simulink model "VCU_CS75_12_27_test_log"  (R2014a)
settings: Solver=FixedStepDiscrete  StartTime=0.0  StopTime=25  FixedStep=0.0005  RelTol=1e-3
undefined symbols (not defined in the file or in its folder): ecucoder_acal, ErrorSumMax1, ErrorSumMax2, ErrorSumMax3, I1, I2, I3, I_SW01_L, LaterlAngleCommand, LDW, Log_ErrorSumMax1, Log_ErrorSumMax2, Log_I1, Log_I2, Log_P1, Log_P2, Log_Takeover, P1, P2, P3, RemoteAcc, RemoteAcclPosition
libraries: simulink x927, ec5744lib x40
(part 2 of 31)

== system VCU_CS75_12_27_test_log/长安CS75底盘程序，20ms一次/Input/CAN1_Rx/TCU_286 ==
  CANReceive : ec5744lib/RapidECU_U3/04CANCommunication/CANReceive  canmodule=1  canbuffer=22  canmessageid=hex2dec('286')  canmessagetype=Standard(11-bit ID)  datalength=8  sampletime=-1
  ReceiveMessages : Subsystem
  Terminator : Terminator
  Terminator1 : Terminator
  TCU_286 : Outport
  wires:
  ReceiveMessages/1(TCU_286) -> TCU_286/1
  CANReceive/3 -> Terminator/1
  CANReceive/4 -> ReceiveMessages/2(In2)
  CANReceive/1 -> ReceiveMessages/Trigger
  CANReceive/2 -> ReceiveMessages/1(In1)
  CANReceive/5 -> Terminator1/1

== system VCU_CS75_12_27_test_log/长安CS75底盘程序，20ms一次/Input/DBC转化的messages（存底）/ReceiveMessages ==
  EMS_205 : Subsystem
  EMS_205_GND : Ground
  EMS_CheckSum_205_Ter : Terminator
  EMS_ESPTorqReuestAvailability_Ter : Terminator
  EMS_FrictionalTorq_Ter : Terminator
  EMS_IndicatedDriverReqTorq_Ter : Terminator
  EMS_IndicatedRealEngTorq_Ter : Terminator
  EMS_RollingCounter_id205_Ter : Terminator
  EMS_TorqFailure_Ter : Terminator
  wires:
  EMS_205/1(EMS_ESPTorqReuestAvailability_Out) -> EMS_ESPTorqReuestAvailability_Ter/1
  EMS_205/2(EMS_TorqFailure_Out) -> EMS_TorqFailure_Ter/1
  EMS_205/3(EMS_IndicatedDriverReqTorq_Out) -> EMS_IndicatedDriverReqTorq_Ter/1
  EMS_205/4(EMS_FrictionalTorq_Out) -> EMS_FrictionalTorq_Ter/1
  EMS_205/5(EMS_IndicatedRealEngTorq_Out) -> EMS_IndicatedRealEngTorq_Ter/1
  EMS_205/6(EMS_RollingCounter_id205_Out) -> EMS_RollingCounter_id205_Ter/1
  EMS_205/7(EMS_CheckSum_205_Out) -> EMS_CheckSum_205_Ter/1
  EMS_205_GND/1 -> EMS_205/1(input)

== system VCU_CS75_12_27_test_log/长安CS75底盘程序，20ms一次/Input/DBC转化的messages（存底）/ReceiveMessages1 ==
  EMS_255 : Subsystem
  EMS_255_GND : Ground
  EMS_AccPedal_Ter : Terminator
  EMS_AccpedelError_Ter : Terminator
  EMS_BrakePedalStatus_Ter : Terminator
  EMS_CheckSum_255_Ter : Terminator
  EMS_EngineSpeedError_Ter : Terminator
  EMS_EngineSpeed_Ter : Terminator
  EMS_RollingCounter_id255_Ter : Terminator
  wires:
  EMS_255/1(EMS_BrakePedalStatus_Out) -> EMS_BrakePedalStatus_Ter/1
  EMS_255/2(EMS_AccpedelError_Out) -> EMS_AccpedelError_Ter/1
  EMS_255/3(EMS_EngineSpeedError_Out) -> EMS_EngineSpeedError_Ter/1
  EMS_255/4(EMS_EngineSpeed_Out) -> EMS_EngineSpeed_Ter/1
  EMS_255/5(EMS_AccPedal_Out) -> EMS_AccPedal_Ter/1
  EMS_255/6(EMS_RollingCounter_id255_Out) -> EMS_RollingCounter_id255_Ter/1
  EMS_255/7(EMS_CheckSum_255_Out) -> EMS_CheckSum_255_Ter/1
  EMS_255_GND/1 -> EMS_255/1(input)

== system VCU_CS75_12_27_test_log/长安CS75底盘程序，20ms一次/Input/DBC转化的messages（存底）/ReceiveMessages10 ==
  ESP_287 : Subsystem
  ESP_287_GND : Ground
  ESP_CheckSum_Ter : Terminator
  ESP_HBBActiveStatus_Ter : Terminator
  ESP_HBB_Status_Ter : Terminator
  ESP_HDC_Status_Ter : Terminator
  ESP_HHC_Available_Ter : Terminator
  ESP_LatAcceleration_Ter : Terminator
  ESP_LongAccelValid_Ter : Terminator
  ESP_LongAcceleration_Ter : Terminator
  ESP_RollingCounter_Ter : Terminator
  ESP_TODFastOpenRequest_Ter : Terminator
  ESP_TODTorqueMaxLimit_Ter : Terminator
  ESP_YawRate_Status_Ter : Terminator
  ESP_YawRate_Ter : Terminator
  wires:
  ESP_287_GND/1 -> ESP_287/1(input)
  ESP_287/13(ESP_RollingCounter_Out) -> ESP_RollingCounter_Ter/1
  ESP_287/12(ESP_CheckSum_Out) -> ESP_CheckSum_Ter/1
  ESP_287/11(ESP_YawRate_Status_Out) -> ESP_YawRate_Status_Ter/1
  ESP_287/10(ESP_LongAccelValid_Out) -> ESP_LongAccelValid_Ter/1
  ESP_287/9(ESP_HBBActiveStatus_Out) -> ESP_HBBActiveStatus_Ter/1
  ESP_287/8(ESP_HHC_Available_Out) -> ESP_HHC_Available_Ter/1
  ESP_287/7(ESP_HBB_Status_Out) -> ESP_HBB_Status_Ter/1
  ESP_287/6(ESP_YawRate_Out) -> ESP_YawRate_Ter/1
  ESP_287/5(ESP_LongAcceleration_Out) -> ESP_LongAcceleration_Ter/1
  ESP_287/4(ESP_LatAcceleration_Out) -> ESP_LatAcceleration_Ter/1
  ESP_287/3(ESP_TODFastOpenRequest_Out) -> ESP_TODFastOpenRequest_Ter/1
  ESP_287/2(ESP_HDC_Status_Out) -> ESP_HDC_Status_Ter/1
  ESP_287/1(ESP_TODTorqueMaxLimit_Out) -> ESP_TODTorqueMaxLimit_Ter/1

== system VCU_CS75_12_27_test_log/长安CS75底盘程序，20ms一次/Input/DBC转化的messages（存底）/ReceiveMessages11 ==
  HU_AEBOnOffSetting_Ter : Terminator
  HU_AEBSetting_551 : Subsystem
  HU_AEBSetting_551_GND : Ground
  HU_FCWSetting_Ter : Terminator
  HU_LCASetting_Ter : Terminator
  wires:
  HU_AEBSetting_551_GND/1 -> HU_AEBSetting_551/1(input)
  HU_AEBSetting_551/3(HU_FCWSetting_Out) -> HU_FCWSetting_Ter/1
  HU_AEBSetting_551/2(HU_LCASetting_Out) -> HU_LCASetting_Ter/1
  HU_AEBSetting_551/1(HU_AEBOnOffSetting_Out) -> HU_AEBOnOffSetting_Ter/1

== system VCU_CS75_12_27_test_log/长安CS75底盘程序，20ms一次/Input/DBC转化的messages（存底）/ReceiveMessages12 ==
  HU_AudioWarningEnable_Ter : Terminator
  HU_BSD_LCAEnable_Ter : Terminator
  HU_CTAEnable_Ter : Terminator
  HU_DSMMemoryPositionFeedback_Ter : Terminator
  HU_DVRBrowseCommand_Ter : Terminator
  HU_HMAEnable_Ter : Terminator
  HU_IACCEnable_Ter : Terminator
  HU_LASModeSelection_Ter : Terminator
  HU_LASSetting_0x541 : Subsystem
  HU_LASSetting_0x541_GND : Ground
  HU_LASWarningModeSelection_Ter : Terminator
  HU_LCATTCSetting_Ter : Terminator
  HU_LDWShakeLev_Ter : Terminator
  HU_LdwSensitivity_Ter : Terminator
  HU_LockCtrlEnable_Ter : Terminator
  HU_ObstacleSafeDistanceSet_Ter : Terminator
  HU_OverspeedSoundWarEnable_Ter : Terminator
  HU_OverspeedWarningEnable_Ter : Terminator
  HU_OverspeedWarningOffset_Ter : Terminator
  HU_ParkingConfirm_Ter : Terminator
  HU_ParkingResume_Ter : Terminator
  HU_RCWEnable_Ter : Terminator
  HU_RCWSoundEnable_Ter : Terminator
  HU_RemoteDistanceSet_Ter : Terminator
  HU_SEWEnable_Ter : Terminator
  HU_SLASwitch_Ter : Terminator
  HU_Uls_BSD_Activation_Ter : Terminator
  HU_Uls_FKP_Activation_Ter : Terminator
  wires:
  HU_LASSetting_0x541_GND/1 -> HU_LASSetting_0x541/1(input)
  HU_LASSetting_0x541/26(HU_DVRBrowseCommand_Out) -> HU_DVRBrowseCommand_Ter/1
  HU_LASSetting_0x541/25(HU_ObstacleSafeDistanceSet_Out) -> HU_ObstacleSafeDistanceSet_Ter/1
  HU_LASSetting_0x541/24(HU_ParkingConfirm_Out) -> HU_ParkingConfirm_Ter/1
  HU_LASSetting_0x541/23(HU_RemoteDistanceSet_Out) -> HU_RemoteDistanceSet_Ter/1
  HU_LASSetting_0x541/22(HU_DSMMemoryPositionFeedback_Out) -> HU_DSMMemoryPositionFeedback_Ter/1
  HU_LASSetting_0x541/21(HU_ParkingResume_Out) -> HU_ParkingResume_Ter/1
  HU_LASSetting_0x541/20(HU_Uls_FKP_Activation_Out) -> HU_Uls_FKP_Activation_Ter/1
  HU_LASSetting_0x541/19(HU_LCATTCSetting_Out) -> HU_LCATTCSetting_Ter/1
  HU_LASSetting_0x541/18(HU_Uls_BSD_Activation_Out) -> HU_Uls_BSD_Activation_Ter/1
  HU_LASSetting_0x541/17(HU_OverspeedWarningOffset_Out) -> HU_OverspeedWarningOffset_Ter/1
  HU_LASSetting_0x541/16(HU_OverspeedWarningEnable_Out) -> HU_OverspeedWarningEnable_Ter/1
  HU_LASSetting_0x541/15(HU_OverspeedSoundWarEnable_Out) -> HU_OverspeedSoundWarEnable_Ter/1
  HU_LASSetting_0x541/14(HU_IACCEnable_Out) -> HU_IACCEnable_Ter/1
  HU_LASSetting_0x541/13(HU_LockCtrlEnable_Out) -> HU_LockCtrlEnable_Ter/1
  HU_LASSetting_0x541/12(HU_AudioWarningEnable_Out) -> HU_AudioWarningEnable_Ter/1
  HU_LASSetting_0x541/11(HU_LDWShakeLev_Out) -> HU_LDWShakeLev_Ter/1
  HU_LASSetting_0x541/10(HU_RCWSoundEnable_Out) -> HU_RCWSoundEnable_Ter/1
  HU_LASSetting_0x541/9(HU_SEWEnable_Out) -> HU_SEWEnable_Ter/1
  HU_LASSetting_0x541/8(HU_RCWEnable_Out) -> HU_RCWEnable_Ter/1
  HU_LASSetting_0x541/7(HU_HMAEnable_Out) -> HU_HMAEnable_Ter/1
  HU_LASSetting_0x541/6(HU_SLASwitch_Out) -> HU_SLASwitch_Ter/1
  HU_LASSetting_0x541/5(HU_LASWarningModeSelection_Out) -> HU_LASWarningModeSelection_Ter/1
  HU_LASSetting_0x541/4(HU_LdwSensitivity_Out) -> HU_LdwSensitivity_Ter/1
  HU_LASSetting_0x541/3(HU_LASModeSelection_Out) -> HU_LASModeSelection_Ter/1
  HU_LASSetting_0x541/2(HU_BSD_LCAEnable_Out) -> HU_BSD_LCAEnable_Ter/1
  HU_LASSetting_0x541/1(HU_CTAEnable_Out) -> HU_CTAEnable_Ter/1

== system VCU_CS75_12_27_test_log/长安CS75底盘程序，20ms一次/Input/DBC转化的messages（存底）/ReceiveMessages13 ==
  SAS_108 : Subsystem
  SAS_108_GND : Ground
  SAS_CRCCheck_Ter : Terminator
  SAS_Calibrated_Ter : Terminator
  SAS_RollingCounter_Ter : Terminator
  SAS_SASFailure_Ter : Terminator
  SAS_SteeringAngleSpeed_Ter : Terminator
  SAS_SteeringAngleValid_Ter : Terminator
  SAS_SteeringAngle_Ter : Terminator
  wires:
  SAS_108_GND/1 -> SAS_108/1(input)
  SAS_108/7(SAS_CRCCheck_Out) -> SAS_CRCCheck_Ter/1
  SAS_108/6(SAS_RollingCounter_Out) -> SAS_RollingCounter_Ter/1
  SAS_108/5(SAS_SteeringAngleValid_Out) -> SAS_SteeringAngleValid_Ter/1
  SAS_108/4(SAS_SASFailure_Out) -> SAS_SASFailure_Ter/1
  SAS_108/3(SAS_Calibrated_Out) -> SAS_Calibrated_Ter/1
  SAS_108/2(SAS_SteeringAngleSpeed_Out) -> SAS_SteeringAngleSpeed_Ter/1
  SAS_108/1(SAS_SteeringAngle_Out) -> SAS_SteeringAngle_Ter/1

== system VCU_CS75_12_27_test_log/长安CS75底盘程序，20ms一次/Input/DBC转化的messages（存底）/ReceiveMessages14 ==
  SCM_3B8 : Subsystem
  SCM_3B8_GND : Ground
  SCM_ACCCancel_Ter : Terminator
  SCM_ACCOn_Ter : Terminator
  SCM_IACCOn_Ter : Terminator
  SCM_Resume_Ter : Terminator
  SCM_Speeddecrease_Ter : Terminator
  SCM_TimeGap_Ter : Terminator
  wires:
  SCM_3B8_GND/1 -> SCM_3B8/1(input)
  SCM_3B8/6(SCM_IACCOn_Out) -> SCM_IACCOn_Ter/1
  SCM_3B8/5(SCM_TimeGap_Out) -> SCM_TimeGap_Ter/1
  SCM_3B8/4(SCM_Speeddecrease_Out) -> SCM_Speeddecrease_Ter/1
  SCM_3B8/3(SCM_Resume_Out) -> SCM_Resume_Ter/1
  SCM_3B8/2(SCM_ACCCancel_Out) -> SCM_ACCCancel_Ter/1
  SCM_3B8/1(SCM_ACCOn_Out) -> SCM_ACCOn_Ter/1

== system VCU_CS75_12_27_test_log/长安CS75底盘程序，20ms一次/Input/DBC转化的messages（存底）/ReceiveMessages15 ==
  SRS_005 : Subsystem
  SRS_005_GND : Ground
  SRS_DriverBuckleSwitchStatus_Ter : Terminator
  SRS_RollingCounter_Ter : Terminator
  wires:
  SRS_005_GND/1 -> SRS_005/1(input)
  SRS_005/2(SRS_RollingCounter_Out) -> SRS_RollingCounter_Ter/1
  SRS_005/1(SRS_DriverBuckleSwitchStatus_Out) -> SRS_DriverBuckleSwitchStatus_Ter/1

== system VCU_CS75_12_27_test_log/长安CS75底盘程序，20ms一次/Input/DBC转化的messages（存底）/ReceiveMessages16 ==
  TCU_286 : Subsystem
  TCU_286_GND : Ground
  TCU_ActualGearValid_Ter : Terminator
  TCU_ActualGear_Ter : Terminator
  TCU_GearShiftPosition_Ter : Terminator
  TCU_ShiftPositionValid_Ter : Terminator
  wires:
  TCU_286_GND/1 -> TCU_286/1(input)
  TCU_286/4(TCU_GearShiftPosition_Out) -> TCU_GearShiftPosition_Ter/1
  TCU_286/3(TCU_ActualGearValid_Out) -> TCU_ActualGearValid_Ter/1
  TCU_286/2(TCU_ShiftPositionValid_Out) -> TCU_ShiftPositionValid_Ter/1
  TCU_286/1(TCU_ActualGear_Out) -> TCU_ActualGear_Ter/1

== system VCU_CS75_12_27_test_log/长安CS75底盘程序，20ms一次/Input/DBC转化的messages（存底）/ReceiveMessages17 ==
  BCM_288 : Subsystem
  BCM_288_GND : Ground
  BCM_BuzzerWarningMode_Ter : Terminator
  BCM_DriverDoorLockStatus_Ter : Terminator
  BCM_DriverDoorStatus_Ter : Terminator
  BCM_FrontWashStatus_Ter : Terminator
  BCM_FrontWiperStatus_Ter : Terminator
  BCM_HoodStatus_Ter : Terminator
  BCM_LatchOverheatProtect_Ter : Terminator
  BCM_LeftRearDoorStatus_Ter : Terminator
  BCM_PassengerDoorLockStatus_Ter : Terminator
  BCM_PassengerDoorStatus_Ter : Terminator
  BCM_PowerStatusFeedback_Ter : Terminator
  BCM_RearWiperStatus_Ter : Terminator
  BCM_ReversePosition_Ter : Terminator
  BCM_RightRearDoorStatus_Ter : Terminator
  BCM_SystemFailureFlag_Ter : Terminator
  BCM_TrunkDoorStatus_Ter : Terminator
  BCM_TurnIndicatorLeft_Ter : Terminator
  BCM_TurnIndicatorRight_Ter : Terminator
  BCM_TurnLightSwitchSts_Ter : Terminator
  BCM_emergencylightstatus_Ter : Terminator
  wires:
  BCM_288_GND/1 -> BCM_288/1(input)
  BCM_288/20(BCM_LatchOverheatProtect_Out) -> BCM_LatchOverheatProtect_Ter/1
  BCM_288/19(BCM_SystemFailureFlag_Out) -> BCM_SystemFailureFlag_Ter/1
  BCM_288/18(BCM_BuzzerWarningMode_Out) -> BCM_BuzzerWarningMode_Ter/1
  BCM_288/17(BCM_TurnLightSwitchSts_Out) -> BCM_TurnLightSwitchSts_Ter/1
  BCM_288/16(BCM_ReversePosition_Out) -> BCM_ReversePosition_Ter/1
  BCM_288/15(BCM_FrontWiperStatus_Out) -> BCM_FrontWiperStatus_Ter/1
  BCM_288/14(BCM_RearWiperStatus_Out) -> BCM_RearWiperStatus_Ter/1
  BCM_288/13(BCM_PowerStatusFeedback_Out) -> BCM_PowerStatusFeedback_Ter/1
  BCM_288/12(BCM_DriverDoorLockStatus_Out) -> BCM_DriverDoorLockStatus_Ter/1
  BCM_288/11(BCM_emergencylightstatus_Out) -> BCM_emergencylightstatus_Ter/1
  BCM_288/10(BCM_PassengerDoorLockStatus_Out) -> BCM_PassengerDoorLockStatus_Ter/1
  BCM_288/9(BCM_DriverDoorStatus_Out) -> BCM_DriverDoorStatus_Ter/1
  BCM_288/8(BCM_PassengerDoorStatus_Out) -> BCM_PassengerDoorStatus_Ter/1
  BCM_288/7(BCM_LeftRearDoorStatus_Out) -> BCM_LeftRearDoorStatus_Ter/1
  BCM_288/6(BCM_RightRearDoorStatus_Out) -> BCM_RightRearDoorStatus_Ter/1
  BCM_288/5(BCM_TrunkDoorStatus_Out) -> BCM_TrunkDoorStatus_Ter/1
  BCM_288/4(BCM_HoodStatus_Out) -> BCM_HoodStatus_Ter/1
  BCM_288/3(BCM_TurnIndicatorLeft_Out) -> BCM_TurnIndicatorLeft_Ter/1
  BCM_288/2(BCM_TurnIndicatorRight_Out) -> BCM_TurnIndicatorRight_Ter/1
  BCM_288/1(BCM_FrontWashStatus_Out) -> BCM_FrontWashStatus_Ter/1

== system VCU_CS75_12_27_test_log/长安CS75底盘程序，20ms一次/Input/DBC转化的messages（存底）/ReceiveMessages18 ==
  BCM_328 : Subsystem
  BCM_328_GND : Ground
  LCM_DRLSts_Ter : Terminator
  LCM_DriveMode_Ter : Terminator
  LCM_LASSwitch_Ter : Terminator
  LCM_RearLeftTuningLightFaultSts_Ter : Terminator
  LCM_RearRightTuningLightFaultSts_Ter : Terminator
  LCM_ReverseLightSts_Ter : Terminator
  wires:
  BCM_328_GND/1 -> BCM_328/1(input)
  BCM_328/6(LCM_ReverseLightSts_Out) -> LCM_ReverseLightSts_Ter/1
  BCM_328/5(LCM_RearLeftTuningLightFaultSts_Out) -> LCM_RearLeftTuningLightFaultSts_Ter/1
  BCM_328/4(LCM_RearRightTuningLightFaultSts_Out) -> LCM_RearRightTuningLightFaultSts_Ter/1
  BCM_328/3(LCM_LASSwitch_Out) -> LCM_LASSwitch_Ter/1
  BCM_328/2(LCM_DRLSts_Out) -> LCM_DRLSts_Ter/1
  BCM_328/1(LCM_DriveMode_Out) -> LCM_DriveMode_Ter/1

== system VCU_CS75_12_27_test_log/长安CS75底盘程序，20ms一次/Input/DBC转化的messages（存底）/ReceiveMessages19 ==
  BCM_348 : Subsystem
  BCM_348_GND : Ground
  BCM_DriveMode_Ter : Terminator
  BCM_LockSignal_Ter : Terminator
  BCM_UnlockSignal_Ter : Terminator
  wires:
  BCM_348_GND/1 -> BCM_348/1(input)
  BCM_348/3(BCM_UnlockSignal_Out) -> BCM_UnlockSignal_Ter/1
  BCM_348/2(BCM_LockSignal_Out) -> BCM_LockSignal_Ter/1
  BCM_348/1(BCM_DriveMode_Out) -> BCM_DriveMode_Ter/1

== system VCU_CS75_12_27_test_log/长安CS75底盘程序，20ms一次/Input/DBC转化的messages（存底）/ReceiveMessages2 ==
  EMS_265 : Subsystem
  EMS_265_GND : Ground
  EMS_EngineStatus_Ter : Terminator
  EMS_FullLoadIndicatedTorq_Ter : Terminator
  EMS_RollingCounter_id265_Ter : Terminator
  EMS_TorqueConstant_Ter : Terminator
  wires:
  EMS_265/1(EMS_FullLoadIndicatedTorq_Out) -> EMS_FullLoadIndicatedTorq_Ter/1
  EMS_265/2(EMS_TorqueConstant_Out) -> EMS_TorqueConstant_Ter/1
  EMS_265/3(EMS_RollingCounter_id265_Out) -> EMS_RollingCounter_id265_Ter/1
  EMS_265/4(EMS_EngineStatus_Out) -> EMS_EngineStatus_Ter/1
  EMS_265_GND/1 -> EMS_265/1(input)

== system VCU_CS75_12_27_test_log/长安CS75底盘程序，20ms一次/Input/DBC转化的messages（存底）/ReceiveMessages20 ==
  BCM_3DF : Subsystem
  BCM_3DF_GND : Ground
  BCM_AmbientLightColorFeedback_Ter : Terminator
  BCM_CRC_Checksum_Ter : Terminator
  BCM_DriveModeFeedback_Ter : Terminator
  BCM_DriveModeStatus_Ter : Terminator
  BCM_DriveMode_Ter : Terminator
  BCM_EPSTorqueModeFeedback_Ter : Terminator
  BCM_EPSTorqueMode_Ter : Terminator
  BCM_RollingCounter_Ter : Terminator
  wires:
  BCM_3DF_GND/1 -> BCM_3DF/1(input)
  BCM_3DF/8(BCM_CRC_Checksum_Out) -> BCM_CRC_Checksum_Ter/1
  BCM_3DF/7(BCM_RollingCounter_Out) -> BCM_RollingCounter_Ter/1
  BCM_3DF/6(BCM_AmbientLightColorFeedback_Out) -> BCM_AmbientLightColorFeedback_Ter/1
  BCM_3DF/5(BCM_EPSTorqueModeFeedback_Out) -> BCM_EPSTorqueModeFeedback_Ter/1
  BCM_3DF/4(BCM_DriveModeFeedback_Out) -> BCM_DriveModeFeedback_Ter/1
  BCM_3DF/3(BCM_DriveModeStatus_Out) -> BCM_DriveModeStatus_Ter/1
  BCM_3DF/2(BCM_EPSTorqueMode_Out) -> BCM_EPSTorqueMode_Ter/1
  BCM_3DF/1(BCM_DriveMode_Out) -> BCM_DriveMode_Ter/1

== system VCU_CS75_12_27_test_log/长安CS75底盘程序，20ms一次/Input/DBC转化的messages（存底）/ReceiveMessages21 ==
  EMS_BrakePedalStatus_Ter : Terminator
  EMS_EngineStartupEnd_Ter : Terminator
  EMS_EngineStatus_Ter : Terminator
  EPB_BrakeLightOnRequest_Ter : Terminator
  EPB_Status_Ter : Terminator
  GW_20B : Subsystem
  GW_20B_GND : Ground
  SAS_SteeringAngleValid_Ter : Terminator
  SAS_SteeringAngle_Ter : Terminator
  TCU_GearShiftPositon_Ter : Terminator
  TCU_ShiftPostionValid_Ter : Terminator
  wires:
  GW_20B_GND/1 -> GW_20B/1(input)
  GW_20B/9(EPB_Status_Out) -> EPB_Status_Ter/1
  GW_20B/8(TCU_ShiftPostionValid_Out) -> TCU_ShiftPostionValid_Ter/1
  GW_20B/7(TCU_GearShiftPositon_Out) -> TCU_GearShiftPositon_Ter/1
  GW_20B/6(EPB_BrakeLightOnRequest_Out) -> EPB_BrakeLightOnRequest_Ter/1
  GW_20B/5(SAS_SteeringAngle_Out) -> SAS_SteeringAngle_Ter/1
  GW_20B/4(EMS_EngineStartupEnd_Out) -> EMS_EngineStartupEnd_Ter/1
  GW_20B/3(EMS_BrakePedalStatus_Out) -> EMS_BrakePedalStatus_Ter/1
  GW_20B/2(EMS_EngineStatus_Out) -> EMS_EngineStatus_Ter/1
  GW_20B/1(SAS_SteeringAngleValid_Out) -> SAS_SteeringAngleValid_Ter/1

== system VCU_CS75_12_27_test_log/长安CS75底盘程序，20ms一次/Input/DBC转化的messages（存底）/ReceiveMessages22 ==
  EMS_EngineSpeed_Ter : Terminator
  GW_332 : Subsystem
  GW_332_GND : Ground
  SAS_SASFailure_Ter : Terminator
  SRS_DriverBuckleSwitchStatus_Ter : Terminator
  SRS_PassengerBuckleSwitchStatus_Ter : Terminator
  wires:
  GW_332_GND/1 -> GW_332/1(input)
  GW_332/4(EMS_EngineSpeed_Out) -> EMS_EngineSpeed_Ter/1
  GW_332/3(SAS_SASFailure_Out) -> SAS_SASFailure_Ter/1
  GW_332/2(SRS_DriverBuckleSwitchStatus_Out) -> SRS_DriverBuckleSwitchStatus_Ter/1
  GW_332/1(SRS_PassengerBuckleSwitchStatus_Out) -> SRS_PassengerBuckleSwitchStatus_Ter/1

== system VCU_CS75_12_27_test_log/长安CS75底盘程序，20ms一次/Input/DBC转化的messages（存底）/ReceiveMessages23 ==
  GW_308 : Subsystem
  GW_308_GND : Ground
  IP_TotalOdometer_Ter : Terminator
  wires:
  GW_308_GND/1 -> GW_308/1(input)
  GW_308/1(IP_TotalOdometer_Out) -> IP_TotalOdometer_Ter/1

== system VCU_CS75_12_27_test_log/长安CS75底盘程序，20ms一次/Input/DBC转化的messages（存底）/ReceiveMessages24 ==
  EMS_ConditionIdle_Ter : Terminator
  EMS_EngineFuelCutOff_Ter : Terminator
  EMS_FrictionalTorq_Ter : Terminator
  EMS_TorqueConstant_Ter : Terminator
  GW_376 : Subsystem
  GW_376_GND : Ground
  wires:
  GW_376_GND/1 -> GW_376/1(input)
  GW_376/4(EMS_ConditionIdle_Out) -> EMS_ConditionIdle_Ter/1
  GW_376/3(EMS_EngineFuelCutOff_Out) -> EMS_EngineFuelCutOff_Ter/1
  GW_376/2(EMS_FrictionalTorq_Out) -> EMS_FrictionalTorq_Ter/1
  GW_376/1(EMS_TorqueConstant_Out) -> EMS_TorqueConstant_Ter/1

== system VCU_CS75_12_27_test_log/长安CS75底盘程序，20ms一次/Input/DBC转化的messages（存底）/ReceiveMessages25 ==
  ACC_ACCMode_Ter : Terminator
  EMS_RemindGear_Ter : Terminator
  EMS_RemindShiftGear_Ter : Terminator
  EPB_FunctionLamp_Ter : Terminator
  EPB_SwitchPositionValid_Ter : Terminator
  EPB_SwitchPosition_Ter : Terminator
  EPB_TextDisplay_Ter : Terminator
  EPS_EPSFailed_Ter : Terminator
  EPS_TorqueAssistMode_Ter : Terminator
  ESP_AutoHoldActive_Ter : Terminator
  ESP_AutoHoldAvailable_Ter : Terminator
  ESP_EBDFailStatus_Ter : Terminator
  ESP_ESPActiveStatus_Ter : Terminator
  ESP_ESPFunctionStatus_Ter : Terminator
  ESP_HBBFunctionStatus_Ter : Terminator
  ESP_HDC_STATUS_Ter : Terminator
  ESP_HHC_Active_Ter : Terminator
  ESP_HHC_Available_Ter : Terminator
  GW_3A2 : Subsystem
  GW_3A2_GND : Ground
  SRS_LeftRearBuckleSwitchSts_Ter : Terminator
  SRS_MiddleRearBuckleSwitchSts_Ter : Terminator
  SRS_RightRearBuckleSwitchSts_Ter : Terminator
  TCU_FailureLamp_Ter : Terminator
  TCU_GearForDisplay_Ter : Terminator
  TCU_GearIndication_Ter : Terminator
  TCU_PWRLamp_Ter : Terminator
  TCU_ReqTranTempWarning_Ter : Terminator
  TCU_WNTLamp_Ter : Terminator
  wires:
  GW_3A2_GND/1 -> GW_3A2/1(input)
  GW_3A2/27(EMS_RemindShiftGear_Out) -> EMS_RemindShiftGear_Ter/1
  GW_3A2/26(TCU_ReqTranTempWarning_Out) -> TCU_ReqTranTempWarning_Ter/1
  GW_3A2/25(TCU_GearIndication_Out) -> TCU_GearIndication_Ter/1
  GW_3A2/24(ESP_HBBFunctionStatus_Out) -> ESP_HBBFunctionStatus_Ter/1
  GW_3A2/23(TCU_GearForDisplay_Out) -> TCU_GearForDisplay_Ter/1
  GW_3A2/22(ESP_HHC_Available_Out) -> ESP_HHC_Available_Ter/1
  GW_3A2/21(ESP_AutoHoldActive_Out) -> ESP_AutoHoldActive_Ter/1
  GW_3A2/20(ESP_HHC_Active_Out) -> ESP_HHC_Active_Ter/1
  GW_3A2/19(ESP_AutoHoldAvailable_Out) -> ESP_AutoHoldAvailable_Ter/1
  GW_3A2/18(ESP_HDC_STATUS_Out) -> ESP_HDC_STATUS_Ter/1
  GW_3A2/17(EPB_SwitchPositionValid_Out) -> EPB_SwitchPositionValid_Ter/1
  GW_3A2/16(EPB_SwitchPosition_Out) -> EPB_SwitchPosition_Ter/1
  GW_3A2/15(EPB_FunctionLamp_Out) -> EPB_FunctionLamp_Ter/1
  GW_3A2/14(EPS_EPSFailed_Out) -> EPS_EPSFailed_Ter/1
  GW_3A2/13(ESP_EBDFailStatus_Out) -> ESP_EBDFailStatus_Ter/1
  GW_3A2/12(ESP_ESPFunctionStatus_Out) -> ESP_ESPFunctionStatus_Ter/1
  GW_3A2/11(ESP_ESPActiveStatus_Out) -> ESP_ESPActiveStatus_Ter/1
  GW_3A2/10(EPB_TextDisplay_Out) -> EPB_TextDisplay_Ter/1
  GW_3A2/9(SRS_RightRearBuckleSwitchSts_Out) -> SRS_RightRearBuckleSwitchSts_Ter/1
  GW_3A2/8(SRS_MiddleRearBuckleSwitchSts_Out) -> SRS_MiddleRearBuckleSwitchSts_Ter/1
  GW_3A2/7(SRS_LeftRearBuckleSwitchSts_Out) -> SRS_LeftRearBuckleSwitchSts_Ter/1
  GW_3A2/6(TCU_PWRLamp_Out) -> TCU_PWRLamp_Ter/1
  GW_3A2/5(TCU_WNTLamp_Out) -> TCU_WNTLamp_Ter/1
  GW_3A2/4(ACC_ACCMode_Out) -> ACC_ACCMode_Ter/1
  GW_3A2/3(TCU_FailureLamp_Out) -> TCU_FailureLamp_Ter/1
  GW_3A2/2(EMS_RemindGear_Out) -> EMS_RemindGear_Ter/1
  GW_3A2/1(EPS_TorqueAssistMode_Out) -> EPS_TorqueAssistMode_Ter/1

== system VCU_CS75_12_27_test_log/长安CS75底盘程序，20ms一次/Input/DBC转化的messages（存底）/ReceiveMessages26 ==
  GW_567 : Subsystem
  GW_567_GND : Ground
  HU_Byroad_Ter : Terminator
  HU_EnterTunnelInfo_Ter : Terminator
  HU_NavGuiganceStatus_Ter : Terminator
  HU_TunnelDistance_Ter : Terminator
  HU_TunnelLength_Ter : Terminator
  wires:
  GW_567_GND/1 -> GW_567/1(input)
  GW_567/5(HU_NavGuiganceStatus_Out) -> HU_NavGuiganceStatus_Ter/1
  GW_567/4(HU_Byroad_Out) -> HU_Byroad_Ter/1
  GW_567/3(HU_TunnelLength_Out) -> HU_TunnelLength_Ter/1
  GW_567/2(HU_TunnelDistance_Out) -> HU_TunnelDistance_Ter/1
  GW_567/1(HU_EnterTunnelInfo_Out) -> HU_EnterTunnelInfo_Ter/1

== system VCU_CS75_12_27_test_log/长安CS75底盘程序，20ms一次/Input/DBC转化的messages（存底）/ReceiveMessages27 ==
  GPSCurrentLocationValid_Ter : Terminator
  HU_GPS_500 : Subsystem
  HU_GPS_500_GND : Ground
  wires:
  HU_GPS_500_GND/1 -> HU_GPS_500/1(input)
  HU_GPS_500/1(GPSCurrentLocationValid_Out) -> GPSCurrentLocationValid_Ter/1

== system VCU_CS75_12_27_test_log/长安CS75底盘程序，20ms一次/Input/DBC转化的messages（存底）/ReceiveMessages28 ==
  LAS_36E : Subsystem
  LAS_36E_GND : Ground
  LAS_CheckSum_id36E_Ter : Terminator
  LAS_LaneEquationC1_Ter : Terminator
  LAS_LaneEquationC3_Ter : Terminator
  LAS_LaneEquationStatus_Ter : Terminator
  LAS_RoadCurvatureFar_Ter : Terminator
  LAS_RoadCurvatureNear_Ter : Terminator
  LAS_RollingCounter_id36E_Ter : Terminator
  wires:
  LAS_36E_GND/1 -> LAS_36E/1(input)
  LAS_36E/7(LAS_CheckSum_id36E_Out) -> LAS_CheckSum_id36E_Ter/1
  LAS_36E/6(LAS_LaneEquationStatus_Out) -> LAS_LaneEquationStatus_Ter/1
  LAS_36E/5(LAS_RollingCounter_id36E_Out) -> LAS_RollingCounter_id36E_Ter/1
  LAS_36E/4(LAS_LaneEquationC3_Out) -> LAS_LaneEquationC3_Ter/1
  LAS_36E/3(LAS_LaneEquationC1_Out) -> LAS_LaneEquationC1_Ter/1
  LAS_36E/2(LAS_RoadCurvatureNear_Out) -> LAS_RoadCurvatureNear_Ter/1
  LAS_36E/1(LAS_RoadCurvatureFar_Out) -> LAS_RoadCurvatureFar_Ter/1

== system VCU_CS75_12_27_test_log/长安CS75底盘程序，20ms一次/Input/DBC转化的messages（存底）/ReceiveMessages3 ==
  EMS_276 : Subsystem
  EMS_276_GND : Ground
  EMS_RealAccPedal_Ter : Terminator
  wires:
  EMS_276/1(EMS_RealAccPedal_Out) -> EMS_RealAccPedal_Ter/1
  EMS_276_GND/1 -> EMS_276/1(input)

== system VCU_CS75_12_27_test_log/长安CS75底盘程序，20ms一次/Input/DBC转化的messages（存底）/ReceiveMessages4 ==
  EPB_256 : Subsystem
  EPB_256_GND : Ground
  EPB_Checksum_Ter : Terminator
  EPB_FailStatus_Ter : Terminator
  EPB_FailureLamp_Ter : Terminator
  EPB_FunctionLamp_Ter : Terminator
  EPB_RollingCounter_id256_Ter : Terminator
  EPB_Status_Ter : Terminator
  wires:
  EPB_256/1(EPB_FailStatus_Out) -> EPB_FailStatus_Ter/1
  EPB_256/2(EPB_Status_Out) -> EPB_Status_Ter/1
  EPB_256/3(EPB_FunctionLamp_Out) -> EPB_FunctionLamp_Ter/1
  EPB_256/4(EPB_FailureLamp_Out) -> EPB_FailureLamp_Ter/1
  EPB_256/5(EPB_RollingCounter_id256_Out) -> EPB_RollingCounter_id256_Ter/1
  EPB_256/6(EPB_Checksum_Out) -> EPB_Checksum_Ter/1
  EPB_256_GND/1 -> EPB_256/1(input)

== system VCU_CS75_12_27_test_log/长安CS75底盘程序，20ms一次/Input/DBC转化的messages（存底）/ReceiveMessages5 ==
  EPS_20A : Subsystem
  EPS_20A_GND : Ground
  EPS_APA_AbortFeedback_Ter : Terminator
  EPS_APA_ControlFeedback_Ter : Terminator
  EPS_APA_EpasFailed_Ter : Terminator
  EPS_Checksum_Ter : Terminator
  EPS_ConcussAvailabilityStatus_Ter : Terminator
  EPS_EPSFailed_Ter : Terminator
  EPS_RollingCounter_Ter : Terminator
  EPS_SteeringTorque_Ter : Terminator
  EPS_TorqueSensorStatus_Ter : Terminator
  wires:
  EPS_20A/1(EPS_EPSFailed_Out) -> EPS_EPSFailed_Ter/1
  EPS_20A/2(EPS_APA_EpasFailed_Out) -> EPS_APA_EpasFailed_Ter/1
  EPS_20A/3(EPS_APA_AbortFeedback_Out) -> EPS_APA_AbortFeedback_Ter/1
  EPS_20A/4(EPS_SteeringTorque_Out) -> EPS_SteeringTorque_Ter/1
  EPS_20A/5(EPS_TorqueSensorStatus_Out) -> EPS_TorqueSensorStatus_Ter/1
  EPS_20A/6(EPS_APA_ControlFeedback_Out) -> EPS_APA_ControlFeedback_Ter/1
  EPS_20A/7(EPS_RollingCounter_Out) -> EPS_RollingCounter_Ter/1
  EPS_20A/8(EPS_ConcussAvailabilityStatus_Out) -> EPS_ConcussAvailabilityStatus_Ter/1
  EPS_20A/9(EPS_Checksum_Out) -> EPS_Checksum_Ter/1
  EPS_20A_GND/1 -> EPS_20A/1(input)

== system VCU_CS75_12_27_test_log/长安CS75底盘程序，20ms一次/Input/DBC转化的messages（存底）/ReceiveMessages6 ==
  CRC_Ter : Terminator
  EPS_21A : Subsystem
  EPS_21A_GND : Ground
  EPS_AvailabilityStatus_Ter : Terminator
  EPS_IACC_abortReson_Ter : Terminator
  EPS_MeasTsionBatTorquevalid_Ter : Terminator
  EPS_MeasuredTosionBatTorque_Ter : Terminator
  Rollingcounter_Ter : Terminator
  wires:
  EPS_21A_GND/1 -> EPS_21A/1(input)
  EPS_21A/6(CRC_Out) -> CRC_Ter/1
  EPS_21A/5(Rollingcounter_Out) -> Rollingcounter_Ter/1
  EPS_21A/4(EPS_IACC_abortReson_Out) -> EPS_IACC_abortReson_Ter/1
  EPS_21A/3(EPS_MeasTsionBatTorquevalid_Out) -> EPS_MeasTsionBatTorquevalid_Ter/1
  EPS_21A/2(EPS_AvailabilityStatus_Out) -> EPS_AvailabilityStatus_Ter/1
  EPS_21A/1(EPS_MeasuredTosionBatTorque_Out) -> EPS_MeasuredTosionBatTorque_Ter/1

== system VCU_CS75_12_27_test_log/长安CS75底盘程序，20ms一次/Input/DBC转化的messages（存底）/ReceiveMessages7 ==
  ESP_277 : Subsystem
  ESP_277_GND : Ground
  ESP_ABAactive_Ter : Terminator
  ESP_ABAavailable_Ter : Terminator
  ESP_AEBAvailable_Ter : Terminator
  ESP_AEBdecActive_Ter : Terminator
  ESP_AWBactive_Ter : Terminator
  ESP_AWBavailable_Ter : Terminator
  ESP_BrakeForce_Ter : Terminator
  ESP_BrakeOverHeat_Ter : Terminator
  ESP_CDD_Active_APA_Ter : Terminator
  ESP_CDD_Active_Ter : Terminator
  ESP_CDD_Available_APA_Ter : Terminator
  ESP_CDD_Available_Ter : Terminator
  ESP_CheckSum_277_Ter : Terminator
  ESP_PrefillActive_Ter : Terminator
  ESP_PrefillAvailable_Ter : Terminator
  ESP_RollingCounter_277_Ter : Terminator
  ESP_TCSActive_Ter : Terminator
  ESP_VDCActive_Ter : Terminator
  ESP_VehicleStandstill_Ter : Terminator
  wires:
  ESP_277_GND/1 -> ESP_277/1(input)
  ESP_277/19(ESP_CheckSum_277_Out) -> ESP_CheckSum_277_Ter/1
  ESP_277/18(ESP_RollingCounter_277_Out) -> ESP_RollingCounter_277_Ter/1
  ESP_277/17(ESP_CDD_Available_APA_Out) -> ESP_CDD_Available_APA_Ter/1
  ESP_277/16(ESP_VehicleStandstill_Out) -> ESP_VehicleStandstill_Ter/1
  ESP_277/15(ESP_CDD_Active_APA_Out) -> ESP_CDD_Active_APA_Ter/1
  ESP_277/14(ESP_CDD_Available_Out) -> ESP_CDD_Available_Ter/1
  ESP_277/13(ESP_CDD_Active_Out) -> ESP_CDD_Active_Ter/1
  ESP_277/12(ESP_BrakeOverHeat_Out) -> ESP_BrakeOverHeat_Ter/1
  ESP_277/11(ESP_PrefillActive_Out) -> ESP_PrefillActive_Ter/1
  ESP_277/10(ESP_PrefillAvailable_Out) -> ESP_PrefillAvailable_Ter/1
  ESP_277/9(ESP_ABAactive_Out) -> ESP_ABAactive_Ter/1
  ESP_277/8(ESP_ABAavailable_Out) -> ESP_ABAavailable_Ter/1
  ESP_277/7(ESP_AEBAvailable_Out) -> ESP_AEBAvailable_Ter/1
  ESP_277/6(ESP_AEBdecActive_Out) -> ESP_AEBdecActive_Ter/1
  ESP_277/5(ESP_AWBactive_Out) -> ESP_AWBactive_Ter/1
  ESP_277/4(ESP_AWBavailable_Out) -> ESP_AWBavailable_Ter/1
  ESP_277/3(ESP_TCSActive_Out) -> ESP_TCSActive_Ter/1
  ESP_277/2(ESP_VDCActive_Out) -> ESP_VDCActive_Ter/1
  ESP_277/1(ESP_BrakeForce_Out) -> ESP_BrakeForce_Ter/1

== system VCU_CS75_12_27_test_log/长安CS75底盘程序，20ms一次/Input/DBC转化的messages（存底）/ReceiveMessages8 ==
  ESP_280 : Subsystem
  ESP_280_GND : Ground
  Wheel_Speed_FL_Data_Ter : Terminator
  Wheel_Speed_FL_Direction_Ter : Terminator
  Wheel_Speed_FL_Valid_Data_Ter : Terminator
  Wheel_Speed_FR_Data_Ter : Terminator
  Wheel_Speed_FR_Direction_Ter : Terminator
  Wheel_Speed_FR_Valid_Data_Ter : Terminator
  Wheel_Speed_RL_Data_Ter : Terminator
  Wheel_Speed_RL_Direction_Ter : Terminator
  Wheel_Speed_RL_Valid_Data_Ter : Terminator
  Wheel_Speed_RR_Data_Ter : Terminator
  Wheel_Speed_RR_Direction_Ter : Terminator
  Wheel_Speed_RR_Valid_Data_Ter : Terminator
  wires:
  ESP_280_GND/1 -> ESP_280/1(input)
  ESP_280/12(Wheel_Speed_FL_Valid_Data_Out) -> Wheel_Speed_FL_Valid_Data_Ter/1
  ESP_280/11(Wheel_Speed_FL_Direction_Out) -> Wheel_Speed_FL_Direction_Ter/1
  ESP_280/10(Wheel_Speed_FL_Data_Out) -> Wheel_Speed_FL_Data_Ter/1
  ESP_280/9(Wheel_Speed_FR_Valid_Data_Out) -> Wheel_Speed_FR_Valid_Data_Ter/1
  ESP_280/8(Wheel_Speed_FR_Direction_Out) -> Wheel_Speed_FR_Direction_Ter/1
  ESP_280/7(Wheel_Speed_FR_Data_Out) -> Wheel_Speed_FR_Data_Ter/1
  ESP_280/6(Wheel_Speed_RL_Valid_Data_Out) -> Wheel_Speed_RL_Valid_Data_Ter/1
  ESP_280/5(Wheel_Speed_RL_Direction_Out) -> Wheel_Speed_RL_Direction_Ter/1
  ESP_280/4(Wheel_Speed_RL_Data_Out) -> Wheel_Speed_RL_Data_Ter/1
  ESP_280/3(Wheel_Speed_RR_Valid_Data_Out) -> Wheel_Speed_RR_Valid_Data_Ter/1
  ESP_280/2(Wheel_Speed_RR_Direction_Out) -> Wheel_Speed_RR_Direction_Ter/1
  ESP_280/1(Wheel_Speed_RR_Data_Out) -> Wheel_Speed_RR_Data_Ter/1

== system VCU_CS75_12_27_test_log/长安CS75底盘程序，20ms一次/Input/DBC转化的messages（存底）/ReceiveMessages9 ==
  ESP_281 : Subsystem
  ESP_281_GND : Ground
  ESP_ABSActiveStatus_Ter : Terminator
  ESP_ABSFailStatus_Ter : Terminator
  ESP_BrakePedalStatus_Ter : Terminator
  ESP_Checksum_Ter : Terminator
  ESP_EBDFailStatus_Ter : Terminator
  ESP_ESPActiveStatus_Ter : Terminator
  ESP_ESPFailStatus_Ter : Terminator
  ESP_ESPSwitchStatus_Ter : Terminator
  ESP_RollingCounter_Ter : Terminator
  ESP_VehicleSpeed_Status_Ter : Terminator
  ESP_VehicleSpeed_Ter : Terminator
  wires:
  ESP_281_GND/1 -> ESP_281/1(input)
  ESP_281/11(ESP_Checksum_Out) -> ESP_Checksum_Ter/1
  ESP_281/10(ESP_BrakePedalStatus_Out) -> ESP_BrakePedalStatus_Ter/1
  ESP_281/9(ESP_RollingCounter_Out) -> ESP_RollingCounter_Ter/1
  ESP_281/8(ESP_VehicleSpeed_Status_Out) -> ESP_VehicleSpeed_Status_Ter/1
  ESP_281/7(ESP_VehicleSpeed_Out) -> ESP_VehicleSpeed_Ter/1
  ESP_281/6(ESP_ABSActiveStatus_Out) -> ESP_ABSActiveStatus_Ter/1
  ESP_281/5(ESP_ESPFailStatus_Out) -> ESP_ESPFailStatus_Ter/1
  ESP_281/4(ESP_ABSFailStatus_Out) -> ESP_ABSFailStatus_Ter/1
  ESP_281/3(ESP_EBDFailStatus_Out) -> ESP_EBDFailStatus_Ter/1
  ESP_281/2(ESP_ESPSwitchStatus_Out) -> ESP_ESPSwitchStatus_Ter/1
  ESP_281/1(ESP_ESPActiveStatus_Out) -> ESP_ESPActiveStatus_Ter/1

== system VCU_CS75_12_27_test_log/长安CS75底盘程序，20ms一次/Output/CAN0_Tx/to511 ==
  note: 0~100%
  note: 有效实际扭矩
  note: 摩擦转矩Nm
  note: 发动机持续扭矩/Nm
  note: 满载有效扭矩0~100%
  note: 正负速度-200~200km/h
  note: 弧度
  note: 轮胎转角/度数
  note: 方向盘转角
  note: 正负速度-200~200km/h
  APP_Signals : Inport
  1-D Lookup Table : Lookup_n-D  NumberOfTableDimensions=1  BreakpointsForDimension1=[-500 500]  Table=[-35 35]  InternalRulePriority=Speed  RndMeth=Simplest  InputSameDT=on
  Abs : Abs
  Abs1 : Abs
  Bus Selector : BusSelector  OutputSignals=APP_Input.CAN1_Data_Rx.EMS_205_Data.EMS_FrictionalTorq,APP_Input.CAN1_Data_Rx.EMS_265_Data.EMS_TorqueConstant,APP_Input.CAN1_Data_Rx.EMS_265_Data.EMS_FullLoadIndicatedTorq,APP_Input.CAN1_Data_Rx.EMS_205_Data.EMS_IndicatedRealEngTorq,System_Status.Switch_Status.P6_Value,APP_Input.CAN1_Data_Rx.ESP_280_Data.Wheel_Speed_RL,APP_Input.CAN1_Data_Rx.ESP_280_Data.Wheel_Speed_RR,APP_Input.CAN1_Data_Rx.SAS_108_Data.SAS_SteeringAngle
  CANTransmit : ec5744lib/RapidECU_U3/04CANCommunication/CANTransmit  canmodule=0  canbuffer=8  canmessageid=hex2dec('511')  canmessagetype=Extended(29-bit ID)  datalength=8  sampletime=-1
  Data Type Conversion : DataTypeConversion
  Data Type Conversion1 : DataTypeConversion
  Data Type Conversion2 : DataTypeConversion
  Gain : Gain  Gain=3.1415925/180
  Gain1 : Gain  Gain=0.01
  Terminator{,1..3} (4 alike) : Terminator
  VCU2IPC : Subsystem
  wires:
  APP_Signals/1 -> Bus Selector/1
  VCU2IPC/1(output) -> CANTransmit/1
  CANTransmit/1 -> Terminator/1
  Bus Selector/8 -> VCU2IPC/1(Steering_feedback_in), 1-D Lookup Table/1  "<SAS_SteeringAngle>"
  1-D Lookup Table/1 -> Gain/1
  Gain/1 -> VCU2IPC/7(Steering_Angle_Feedback_in)
  Bus Selector/7 -> Abs/1  "<Wheel_Speed_RR>"
  Abs/1 -> VCU2IPC/6(Wheel_Speed_RR_Feedback_in)
  Bus Selector/6 -> Abs1/1  "<Wheel_Speed_RL>"
  Abs1/1 -> VCU2IPC/5(Wheel_Speed_RL_Feedback_in)
  Bus Selector/5 -> VCU2IPC/4(Res_go_in)  "<P6_Value>"
  Bus Selector/4 -> Gain1/1  "<EMS_IndicatedRealEngTorq>"
  Bus Selector/3 -> Data Type Conversion2/1  "<EMS_FullLoadIndicatedTorq>"
  Gain1/1 -> VCU2IPC/3(Engine_Feedback2_in), VCU2IPC/2(Engine_Feedback_in)  "EMS_IndicatedRealTroq"
  Bus Selector/2 -> Data Type Conversion1/1  "<EMS_TorqueConstant>"
  Bus Selector/1 -> Data Type Conversion/1  "<EMS_FrictionalTorq>"
  Data Type Conversion/1 -> Terminator1/1  "EMS_FrictionalTroq"
  Data Type Conversion1/1 -> Terminator2/1  "EMS_TorqueConstant"
  Data Type Conversion2/1 -> Terminator3/1  "EMS_FullLoadIndicatedTroq"

== system VCU_CS75_12_27_test_log/长安CS75底盘程序，20ms一次/Output/CAN0_Tx/to6001 ==
  note: 0是前进
      | 1后退
      | 2parkIng
  APP_Signals : Inport
  A : Subsystem
  Bus Selector : BusSelector  OutputSignals=APP_Input.CAN1_Data_Rx.ESP_280_Data.Wheel_Speed_RR,APP_Input.CAN1_Data_Rx.ESP_280_Data.Wheel_Speed_RR_Direction,APP_Input.CAN1_Data_Rx.ESP_280_Data.Wheel_Speed_RL,APP_Input.CAN1_Data_Rx.ESP_280_Data.Wheel_Speed_RL_Direction,APP_Input.CAN1_Data_Rx.ESP_280_Data.Wheel_Speed_FR,APP_Input.CAN1_Data_Rx.ESP_280_Data.Wheel_Speed_FR_Direction,APP_Input.CAN1_Data_Rx.ESP_280_Data.Wheel_Speed_FL,APP_Input.CAN1_Data_Rx.ESP_280_Data.Wheel_Speed_FL_Direction
  CANTransmit : ec5744lib/RapidECU_U3/04CANCommunication/CANTransmit  canmodule=0  canbuffer=8  canmessageid=hex2dec('6001')  canmessagetype=Extended(29-bit ID)  datalength=8  sampletime=-1
  MATLAB Function : MATLAB Function  TreatAsAtomicUnit=on
  MATLAB Function1 : MATLAB Function  TreatAsAtomicUnit=on
  MATLAB Function2 : MATLAB Function  TreatAsAtomicUnit=on
  MATLAB Function3 : MATLAB Function  TreatAsAtomicUnit=on
  Terminator : Terminator
  wires:
  APP_Signals/1 -> Bus Selector/1
  A/1(output) -> CANTransmit/1
  CANTransmit/1 -> Terminator/1
  MATLAB Function3/1(y) -> A/4(Wheel_Speed_FL_Data_in)
  MATLAB Function2/1(y) -> A/3(Wheel_Speed_FR_Data_in)
  MATLAB Function1/1(y) -> A/2(Wheel_Speed_RL_Data_in)
  MATLAB Function/1(y) -> A/1(Wheel_Speed_RR_Data_in)
  Bus Selector/1 -> MATLAB Function/1(u1)  "<Wheel_Speed_RR>"
  Bus Selector/2 -> MATLAB Function/2(u2)  "<Wheel_Speed_RR_Direction>"
  Bus Selector/3 -> MATLAB Function1/1(u1)  "<Wheel_Speed_RL>"
  Bus Selector/4 -> MATLAB Function1/2(u2)  "<Wheel_Speed_RL_Direction>"
  Bus Selector/5 -> MATLAB Function2/1(u1)  "<Wheel_Speed_FR>"
  Bus Selector/6 -> MATLAB Function2/2(u2)  "<Wheel_Speed_FR_Direction>"
  Bus Selector/7 -> MATLAB Function3/1(u1)  "<Wheel_Speed_FL>"
  Bus Selector/8 -> MATLAB Function3/2(u2)  "<Wheel_Speed_FL_Direction>"

== system VCU_CS75_12_27_test_log/长安CS75底盘程序，20ms一次/Output/CAN0_Tx/to6002 ==
  APP_Signals : Inport
  B : Subsystem
  Bus Selector : BusSelector  OutputSignals=Control_Output.Longitudinal_Output.2E4.ACC_ACCTargetAcceleration,APP_Input.CAN1_Data_Rx.EMS_255_Data.EMS_BrakePedalStatus,APP_Input.CAN1_Data_Rx.EMS_276_Data.EMS_RealAccPedal,APP_Input.CAN1_Data_Rx.SAS_108_Data.SAS_SteeringAngle,APP_Input.CAN1_Data_Rx.ESP_281_Data.ESP_VehicleSpeed
  CANTransmit : ec5744lib/RapidECU_U3/04CANCommunication/CANTransmit  canmodule=0  canbuffer=9  canmessageid=hex2dec('6002')  canmessagetype=Extended(29-bit ID)  datalength=8  sampletime=-1
  MATLAB Function : MATLAB Function  TreatAsAtomicUnit=on
  Terminator : Terminator
  wires:
  CANTransmit/1 -> Terminator/1
  B/1(output) -> CANTransmit/1
  APP_Signals/1 -> Bus Selector/1
  Bus Selector/5 -> B/6(VehicleSpeed_in)  "<ESP_VehicleSpeed>"
  Bus Selector/4 -> B/5(Steering_Angle_in)  "<SAS_SteeringAngle>"
  Bus Selector/3 -> B/4(ThrottlePedalPercentage_in)  "<EMS_RealAccPedal>"
  Bus Selector/2 -> B/3(BrakePeadlState_in)  "<EMS_BrakePedalStatus>"
  Bus Selector/1 -> MATLAB Function/1(u)  "<ACC_ACCTargetAcceleration>"
  MATLAB Function/2(y2) -> B/2(RemoteThrottlePercentage_in)
  MATLAB Function/1(y1) -> B/1(RemoteDecelerationRequest_in)

== system VCU_CS75_12_27_test_log/长安CS75底盘程序，20ms一次/Output/CAN0_Tx/to6003 ==
  APP_Signals : Inport
  Bus Selector : BusSelector  OutputSignals=APP_Input.CAN1_Data_Rx.ESP_287_Data.ESP_LongAcceleration,APP_Input.CAN1_Data_Rx.ESP_287_Data.ESP_LatAcceleration,APP_Input.CAN1_Data_Rx.ESP_287_Data.ESP_YawRate
  C : Subsystem
  CANTransmit : ec5744lib/RapidECU_U3/04CANCommunication/CANTransmit  canmodule=0  canbuffer=10  canmessageid=hex2dec('6003')  canmessagetype=Extended(29-bit ID)  datalength=8  sampletime=-1
  Terminator : Terminator
  wires:
  APP_Signals/1 -> Bus Selector/1
  C/1(output) -> CANTransmit/1
  CANTransmit/1 -> Terminator/1
  Bus Selector/3 -> C/3(YawRate_in)  "<ESP_YawRate>"
  Bus Selector/2 -> C/2(LateralAcceleration_in)  "<ESP_LatAcceleration>"
  Bus Selector/1 -> C/1(LongitudinalAcceleration_in)  "<ESP_LongAcceleration>"

== system VCU_CS75_12_27_test_log/长安CS75底盘程序，20ms一次/Output/CAN0_Tx/to6004 ==
  APP_Signals : Inport
  Add : Sum
  Bus Selector : BusSelector  OutputSignals=System_Status.ServerStatus.AutoDrivingReady,System_Status.VehicleStatus.EPS_AvailabilityStatus,System_State,System_Status.ServerStatus.Server_CommunicationStatus,System_Status.VehicleStatus.VehicleCommunicationStatus,APP_Input.CAN0_Data_Rx.A1_Data.LaterlAngleCommand,APP_Input.CAN0_Data_Rx.A1_Data.RemoteAcclPosition
  CANTransmit : ec5744lib/RapidECU_U3/04CANCommunication/CANTransmit  canmodule=0  canbuffer=11  canmessageid=hex2dec('6004')  canmessagetype=Extended(29-bit ID)  datalength=8  sampletime=-1
  D : Subsystem
  Gain : Gain  Gain=2
  MATLAB Function : MATLAB Function  TreatAsAtomicUnit=on
  Terminator : Terminator
  wires:
  CANTransmit/1 -> Terminator/1
  APP_Signals/1 -> Bus Selector/1
  D/1(output) -> CANTransmit/1
  Bus Selector/7 -> D/6(Command_ACC_in)  "<RemoteAcclPosition>"
  Bus Selector/6 -> D/5(CommandSteering_in)  "<LaterlAngleCommand>"
  Bus Selector/5 -> Gain/1  "<VehicleCommunicationStatus>"
  Bus Selector/4 -> Add/1  "<Server_CommunicationStatus>"
  Gain/1 -> Add/2
  Add/1 -> D/4(ControllerErrorState_in)
  Bus Selector/3 -> D/3(FSM_CurrentState_in)  "<System_State>"
  Bus Selector/2 -> MATLAB Function/1(u)  "<EPS_AvailabilityStatus>"
  Bus Selector/1 -> D/1(LongitudinalAutoDrivingState_in)  "<AutoDrivingReady>"
  MATLAB Function/1(y) -> D/2(LateralAutoDrivingSwitch_in)

== system VCU_CS75_12_27_test_log/长安CS75底盘程序，20ms一次/Output/CAN0_Tx/to601 ==
  APP_Signals : Inport
  Bus Selector : BusSelector  OutputSignals=Control_Output.Lateral_Output.SteeringTorqueOut,Control_Output.Lateral_Output.ErrorSum,Control_Output.Lateral_Output.Error
  CANTransmit : ec5744lib/RapidECU_U3/04CANCommunication/CANTransmit  canmodule=0  canbuffer=11  canmessageid=hex2dec('601')  canmessagetype=Standard(11-bit ID)  datalength=8  sampletime=-1
  Message1 : Subsystem
  Terminator : Terminator
  wires:
  APP_Signals/1 -> Bus Selector/1
  Message1/1(output) -> CANTransmit/1
  CANTransmit/1 -> Terminator/1
  Bus Selector/1 -> Message1/3(PID_ST_Out_in)  "<SteeringTorqueOut>"
  Bus Selector/2 -> Message1/2(ErrorSum_in)  "<ErrorSum>"
  Bus Selector/3 -> Message1/1(Error_in)  "<Error>"

== system VCU_CS75_12_27_test_log/长安CS75底盘程序，20ms一次/Output/CAN1_Tx/to28D ==
  APP_Signals : Inport
  Bus Selector : BusSelector  OutputSignals=Control_Output.Accesories_Output.LAS_LDWStatus,Control_Output.Accesories_Output.LAS_LDWVibrationWarning,Control_Output.Lateral_Output.LAS_SteeringTorque,Control_Output.Lateral_Output.LAS_LKSStatus,Control_Output.Lateral_Output.LAS_RollingCounter
  CANTransmit : ec5744lib/RapidECU_U3/04CANCommunication/CANTransmit  canmodule=1  canbuffer=13  canmessageid=hex2dec('28D')  canmessagetype=Standard(11-bit ID)  datalength=8  sampletime=-1
  Constant{,1..7,9,11} (10 alike) : Constant  Value=0
  LAS_28D : Subsystem
  Terminator : Terminator
  wires:
  CANTransmit/1 -> Terminator/1
  LAS_28D/1(output) -> CANTransmit/1
  APP_Signals/1 -> Bus Selector/1
  Bus Selector/5 -> LAS_28D/14(RollingConter_in)  "<LAS_RollingCounter>"
  Bus Selector/2 -> LAS_28D/6(LAS_LDWVibrationWarning_in)  "<LAS_LDWVibrationWarning>"
  Bus Selector/1 -> LAS_28D/2(LAS_LDWStatus_in)  "<LAS_LDWStatus>"
  Constant/1 -> LAS_28D/1(LAS_SLASpdLimitUnit_in)
  Constant1/1 -> LAS_28D/3(LAS_CaliStatus_in)
  Constant2/1 -> LAS_28D/4(LAS_TakeoverReq_in)
  Constant3/1 -> LAS_28D/5(LAS_DFDFailed_in)
  Constant4/1 -> LAS_28D/7(LAS_SLASpdLimit_in)
  Constant5/1 -> LAS_28D/8(LAS_LDWReminder_in)
  Constant6/1 -> LAS_28D/9(LAS_DFDWarning_in)
  Constant7/1 -> LAS_28D/10(LAS_LASFailed_in)
  Constant9/1 -> LAS_28D/12(LAS_SLAState_in)
  Bus Selector/4 -> LAS_28D/13(LAS_LKSStatus_in)  "<LAS_LKSStatus>"
  Constant11/1 -> LAS_28D/15(CRC_in)
  Bus Selector/3 -> LAS_28D/11(LAS_SteeringTorqueReq_in)  "<LAS_SteeringTorque>"

== system VCU_CS75_12_27_test_log/长安CS75底盘程序，20ms一次/Output/CAN1_Tx/to2E4 ==
  APP_Signals : Inport
  ACC_2E4 : Subsystem
  Bus Selector : BusSelector  OutputSignals=Control_Output.Longitudinal_Output.2E4.ACC_CDDAxEnable,Control_Output.Longitudinal_Output.2E4.ACC_DecToStop,Control_Output.Longitudinal_Output.2E4.ACC_Driveoff_Request,Control_Output.Longitudinal_Output.2E4.ACC_Mode,Control_Output.Longitudinal_Output.2E4.ACC_ACCTargetAcceleration,Control_Output.Longitudinal_Output.2E4.ACC_RollingCounter_id2E4
  CANTransmit : ec5744lib/RapidECU_U3/04CANCommunication/CANTransmit  canmodule=1  canbuffer=8  canmessageid=hex2dec('2E4')  canmessagetype=Standard(11-bit ID)  datalength=8  sampletime=-1
  Constant : Constant  Value=0
  Terminator : Terminator
  wires:
  APP_Signals/1 -> Bus Selector/1
  Bus Selector/1 -> ACC_2E4/1(ACC_CDDAxEnable_in)  "<ACC_CDDAxEnable>"
  Bus Selector/2 -> ACC_2E4/2(ACC_DecToStop_in)  "<ACC_DecToStop>"
  Bus Selector/3 -> ACC_2E4/3(ACC_Driveoff_Request_in)  "<ACC_Driveoff_Request>"
  Bus Selector/4 -> ACC_2E4/4(ACC_Mode_in)  "<ACC_Mode>"
  Bus Selector/5 -> ACC_2E4/5(ACC_ACCTargetAcceleration_in)  "<ACC_ACCTargetAcceleration>"
  Bus Selector/6 -> ACC_2E4/6(ACC_RollingCounter_id_in)  "<ACC_RollingCounter_id2E4>"
  Constant/1 -> ACC_2E4/7(ACC_CheckSum_id_in)  "ACC_CheckSum_id"
  ACC_2E4/1(output) -> CANTransmit/1
  CANTransmit/1 -> Terminator/1

== system VCU_CS75_12_27_test_log/长安CS75底盘程序，20ms一次/Output/CAN1_Tx/to2E5 ==
  APP_Signals : Inport
  ACC_2E5 : Subsystem
  Bus Selector : BusSelector  OutputSignals=Control_Output.Longitudinal_Output.2E5.ACC_TrqEnable,Control_Output.Longitudinal_Output.2E5.ACC_AccTorqueReq,Control_Output.Longitudinal_Output.2E5.ACC_RollingCounter_id2E5
  CANTransmit : ec5744lib/RapidECU_U3/04CANCommunication/CANTransmit  canmodule=1  canbuffer=9  canmessageid=hex2dec('2E5')  canmessagetype=Standard(11-bit ID)  datalength=8  sampletime=-1
  Constant{,1..12} (13 alike) : Constant  Value=0
  Terminator : Terminator
  wires:
  CANTransmit/1 -> Terminator/1
  ACC_2E5/1(output) -> CANTransmit/1
  APP_Signals/1 -> Bus Selector/1
  Constant12/1 -> ACC_2E5/1(ACC_AEBTargetDeceleration_in)
  Bus Selector/2 -> ACC_2E5/11(ACC_AccTorqueReq_in)  "<ACC_AccTorqueReq>"
  Constant/1 -> ACC_2E5/16(ACC_CheckSum_in)
  Bus Selector/3 -> ACC_2E5/15(ACC_RollingCounter_in)  "<ACC_RollingCounter_id2E5>"
  Bus Selector/1 -> ACC_2E5/2(ACC_AccTrqReqEnable_in)  "<ACC_TrqEnable>"
  Constant1/1 -> ACC_2E5/14(ACC_TextInfoForDriver_in)
  Constant2/1 -> ACC_2E5/13(ACC_AEBDecCtrlAvail_in)
  Constant3/1 -> ACC_2E5/12(ACC_ABAlevel_in)
  Constant4/1 -> ACC_2E5/10(ACC_AWBavailable_in)
  Constant5/1 -> ACC_2E5/9(ACC_ESPPrefill_in)
  Constant6/1 -> ACC_2E5/8(ACC_PCWPenable_in)
  Constant7/1 -> ACC_2E5/7(ACC_PCW_LatentWarning_in)
  Constant8/1 -> ACC_2E5/6(ACC_PCWPreWarning_in)
  Constant9/1 -> ACC_2E5/5(ACC_AEBLVehilcehold_in)
  Constant10/1 -> ACC_2E5/4(ACC_ABAavailable_in)
  Constant11/1 -> ACC_2E5/3(ACC_AWBlevel_in)

== system VCU_CS75_12_27_test_log/长安CS75底盘程序，20ms一次/Output/CAN1_Tx/to602 ==
  APP_Signals : Inport
  Bus Selector : BusSelector  OutputSignals=APP_Input.CAN0_Data_Rx.A1_Data.RemoteAcclPosition,Control_Output.Longitudinal_Output.Error_Log,Control_Output.Longitudinal_Output.ErrorSum_Log
  CANTransmit : ec5744lib/RapidECU_U3/04CANCommunication/CANTransmit  canmodule=1  canbuffer=60  canmessageid=hex2dec('602')  canmessagetype=Standard(11-bit ID)  datalength=8  sampletime=-1
  Message602 : Subsystem
  Terminator : Terminator
  wires:
  APP_Signals/1 -> Bus Selector/1
  Message602/1(output) -> CANTransmit/1
  CANTransmit/1 -> Terminator/1
  Bus Selector/1 -> Message602/3(RemoteAcc_in)  "<RemoteAcclPosition>"
  Bus Selector/2 -> Message602/2(Error_Log_in)  "<Error_Log>"
  Bus Selector/3 -> Message602/1(ErrorSum_Log_in)  "<ErrorSum_Log>"

== system VCU_CS75_12_27_test_log/长安CS75底盘程序，20ms一次/Output/Subsystem/28A ==
  APA_28A : Subsystem
  APA_28A_Ter : Terminator
  APA_CheckSum : Ground
  APA_EPSAngleReq : Ground
  APA_IncreasePressureReq : Ground
  APA_Indication : Ground
  APA_OnOff : Ground
  APA_RollingCounter : Ground
  APA_SteeringAngleReqProtection : Ground
  wires:
  APA_28A/1(output) -> APA_28A_Ter/1
  APA_CheckSum/1 -> APA_28A/7(APA_CheckSum_in)
  APA_RollingCounter/1 -> APA_28A/6(APA_RollingCounter_in)
  APA_IncreasePressureReq/1 -> APA_28A/5(APA_IncreasePressureReq_in)
  APA_OnOff/1 -> APA_28A/4(APA_OnOff_in)
  APA_Indication/1 -> APA_28A/3(APA_Indication_in)
  APA_EPSAngleReq/1 -> APA_28A/2(APA_EPSAngleReq_in)
  APA_SteeringAngleReqProtection/1 -> APA_28A/1(APA_SteeringAngleReqProtection_in)

== system VCU_CS75_12_27_test_log/长安CS75底盘程序，20ms一次/Output/Subsystem/28D ==
  CRC : Ground
  LAS_28D : Subsystem
  LAS_28D_Ter : Terminator
  LAS_CaliStatus : Ground
  LAS_DFDFailed : Ground
  LAS_DFDWarning : Ground
  LAS_LASFailed : Ground
  LAS_LDWReminder : Ground
  LAS_LDWStatus : Ground
  LAS_LDWVibrationWarning : Ground
  LAS_LKSStatus : Ground
  LAS_SLASpdLimit : Ground
  LAS_SLASpdLimitUnit : Ground
  LAS_SLAState : Ground
  LAS_SteeringTorqueReq : Ground
  LAS_TakeoverReq : Ground
  RollingConter : Ground
  wires:
  LAS_SLASpdLimitUnit/1 -> LAS_28D/1(LAS_SLASpdLimitUnit_in)
  LAS_LDWStatus/1 -> LAS_28D/2(LAS_LDWStatus_in)
  LAS_CaliStatus/1 -> LAS_28D/3(LAS_CaliStatus_in)
  LAS_TakeoverReq/1 -> LAS_28D/4(LAS_TakeoverReq_in)
  LAS_DFDFailed/1 -> LAS_28D/5(LAS_DFDFailed_in)
  LAS_LDWVibrationWarning/1 -> LAS_28D/6(LAS_LDWVibrationWarning_in)
  LAS_SLASpdLimit/1 -> LAS_28D/7(LAS_SLASpdLimit_in)
  LAS_LDWReminder/1 -> LAS_28D/8(LAS_LDWReminder_in)
  LAS_DFDWarning/1 -> LAS_28D/9(LAS_DFDWarning_in)
  LAS_LASFailed/1 -> LAS_28D/10(LAS_LASFailed_in)
  LAS_SteeringTorqueReq/1 -> LAS_28D/11(LAS_SteeringTorqueReq_in)
  LAS_SLAState/1 -> LAS_28D/12(LAS_SLAState_in)
  LAS_LKSStatus/1 -> LAS_28D/13(LAS_LKSStatus_in)
  RollingConter/1 -> LAS_28D/14(RollingConter_in)
  CRC/1 -> LAS_28D/15(CRC_in)
  LAS_28D/1(output) -> LAS_28D_Ter/1

== system VCU_CS75_12_27_test_log/长安CS75底盘程序，20ms一次/Output/Subsystem/2E4 ==
  ACC_2E4 : Subsystem
  ACC_2E4_Ter : Terminator
  ACC_ACCTargetAcceleration : Ground
  ACC_CDDAxEnable : Ground
  ACC_CheckSum_id : Ground
  ACC_DecToStop : Ground
  ACC_Driveoff_Request : Ground
  ACC_Mode : Ground
  ACC_RollingCounter_id : Ground
  wires:
  ACC_CDDAxEnable/1 -> ACC_2E4/1(ACC_CDDAxEnable_in)
  ACC_DecToStop/1 -> ACC_2E4/2(ACC_DecToStop_in)
  ACC_Driveoff_Request/1 -> ACC_2E4/3(ACC_Driveoff_Request_in)
  ACC_Mode/1 -> ACC_2E4/4(ACC_Mode_in)
  ACC_ACCTargetAcceleration/1 -> ACC_2E4/5(ACC_ACCTargetAcceleration_in)
  ACC_RollingCounter_id/1 -> ACC_2E4/6(ACC_RollingCounter_id_in)
  ACC_CheckSum_id/1 -> ACC_2E4/7(ACC_CheckSum_id_in)
  ACC_2E4/1(output) -> ACC_2E4_Ter/1
